simulink model "simlin2"  (R2016a)
settings: Solver=ode4  StartTime=0.0  StopTime=10.0  FixedStep=0.01  RelTol=1e-3
values from neighbouring files (symbols this model uses):
  Ac = eval(subs(Alin,[x1 x2 x3 x4 u],[xlin ulin]))    [linearizacia.m]    (also in linearnySM.mat = [0 0 0 0 1 0 0 0 0 -1.962 0 -58.86 ... (16 elements, 4x4)]; linearnySM2.mat = [0 0 0 0 1 0 0 0 0 -1.962 0 58.86 ... (16 elements, 4x4)]; sysd.mat = [0 0 0 0 1 0 0 0 0 -1.962 0 -58.86 ... (16 elements, 4x4)]; sysd2.mat = [0 0 0 0 1 0 0 0 0 -1.962 0 58.86 ... (16 elements, 4x4)])
  Bc = eval(subs(Blin,[x1 x2 x3 x4 u],[xlin ulin]))    [linearizacia.m]    (also in linearnySM.mat = [0 2.5 0 12.5]; linearnySM2.mat = [0 2.5 0 -12.5]; sysd.mat = [0 2.5 0 12.5]; sysd2.mat = [0 2.5 0 -12.5])
  Cc = eval(subs(Clin,[x1 x2 x3 x4],xlin))    [linearizacia.m]    (also in linearnySM.mat = [1  0  0  0; 0  0  1  0]; linearnySM2.mat = [1  0  0  0; 0  0  1  0]; sysd.mat = [1  0  0  0; 0  0  1  0]; sysd2.mat = [1  0  0  0; 0  0  1  0])
  Dc = eval(subs(Dlin,[x1 x2 x3 x4],xlin))    [linearizacia.m]    (also in linearnySM.mat = [0 0]; linearnySM2.mat = [0 0]; sysd.mat = [0 0]; sysd2.mat = [0 0])
  dx0 = x0-xlin    [kalmankyvadlo.m]    (also in simEKFkyvadlo.m; simKFkyvadlo.m = zeros(nx,1); simdiskkyvadlo.m = [0;0;0;0]; simlinkyvadlo.m = [0;0;-pi/6;0])
settings Model: Creator=gulan  LastModifiedBy=gulan

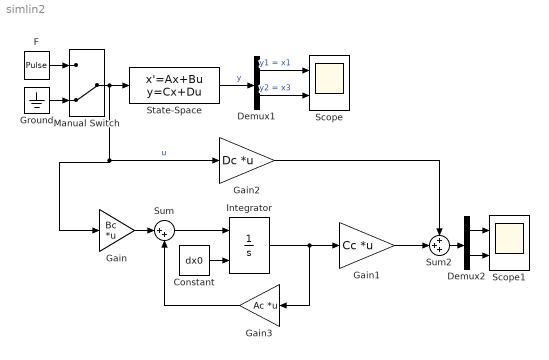
== system simlin2 ==
  " Scope" : Scope  NumInputPorts=2
  " Scope1" : Scope  NumInputPorts=2
  Constant : Constant  Value=dx0  SampleTime=0.01
  Demux1 : Demux  Outputs=2
  Demux2 : Demux  Outputs=2
  F : DiscretePulseGenerator  PulseType=Time based  Amplitude=-1  Period=10  PulseWidth=0.1  PhaseDelay=0.01
  Gain : Gain  Gain=Bc  Multiplication=Matrix(K*u)
  Gain1 : Gain  Gain=Cc  Multiplication=Matrix(K*u) (u vector)
  Gain2 : Gain  Gain=Dc  Multiplication=Matrix(K*u) (u vector)
  Gain3 : Gain  Gain=Ac  Multiplication=Matrix(K*u)
  Ground : Ground
  Integrator : Integrator  InitialConditionSource=external
  Manual Switch : ManualSwitch  CurrentSetting=0
  State-Space : StateSpace  A=Ac  B=Bc  C=Cc  D=Dc  X0=[0;0;-pi/6;0]
  Sum : Sum  Inputs=|++
  Sum2 : Sum  Inputs=+++
  wires:
  State-Space/1 -> Demux1/1  "y"
  F/1 -> Manual Switch/1
  Ground/1 -> Manual Switch/2
  Manual Switch/1 -> Gain/1, Gain2/1, State-Space/1  "u"
  Demux1/1 -> " Scope"/1  "y1 = x1"
  Demux1/2 -> " Scope"/2  "y2 = x3"
  Gain3/1 -> Sum/2
  Gain/1 -> Sum/1
  Sum/1 -> Integrator/1
  Constant/1 -> Integrator/2
  Integrator/1 -> Gain1/1, Gain3/1
  Gain1/1 -> Sum2/2
  Sum2/1 -> Demux2/1
  Demux2/1 -> " Scope1"/1
  Demux2/2 -> " Scope1"/2
  Gain2/1 -> Sum2/1
